simulink model "Sliding_Mode_Control_car"  (R2022b)
settings: Solver=VariableStepAuto  StartTime=0.0  StopTime=30  RelTol=1e-3
undefined symbols (not defined in the file): tao
settings Model: Creator=Miakho  LastModifiedBy=Miakho

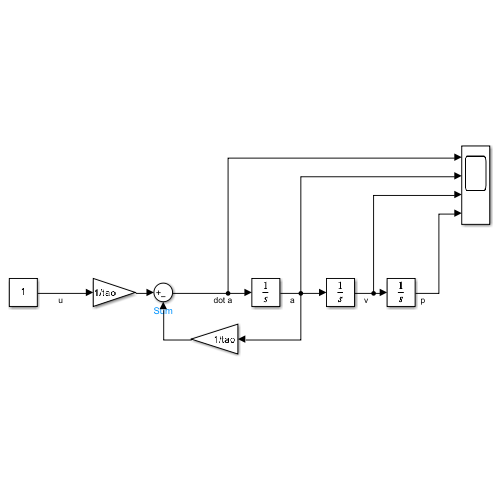
[thumbnail: Simulink's stored preview of the top-level diagram]
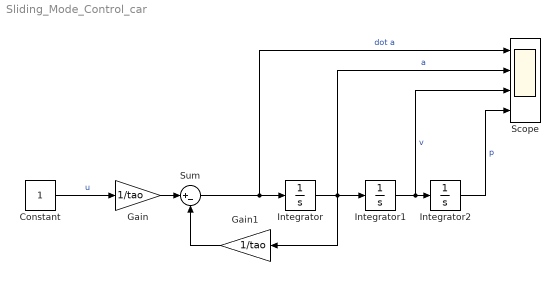
== system Sliding_Mode_Control_car ==
  Constant : Constant
  Gain : Gain  Gain=1/tao
  Gain1 : Gain  Gain=1/tao
  Integrator : Integrator
  Integrator1 : Integrator
  Integrator2 : Integrator
  Scope : Scope  NumInputPorts=4
  Sum : Sum  Inputs=|+-
  wires:
  Integrator/1 -> Scope/2, Gain1/1, Integrator1/1  "a"
  Integrator1/1 -> Scope/3, Integrator2/1  "v"
  Sum/1 -> Scope/1, Integrator/1  "dot a"
  Constant/1 -> Gain/1  "u"
  Gain/1 -> Sum/1
  Gain1/1 -> Sum/2
  Integrator2/1 -> Scope/4  "p"
